simulink model "week1problem8"  (R2020a)
settings: Solver=VariableStepAuto  StartTime=0.0  StopTime=10.0  RelTol=1e-3
settings Model: Creator=Admin  LastModifiedBy=Admin

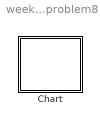
== system week1problem8 ==
  Chart : Stateflow chart  TreatAsAtomicUnit=on

== stateflow chart week1problem8/Chart ==
  state LiftOperation [parallel]
    entry:
    status=0;
    settings: executionOrder=1
    state LiftFunctionOn
      (history)
      state GroundFloor
        entry:
        status=1;
        during:
        CurrentFloor=0;
        FloorCheck(CurrentFloor);
        exit:
        status=0;
      state FirstFloor
        entry:
        status=1;
        during:
        CurrentFloor=1;
        FloorCheck(CurrentFloor);
        exit:
        status=0;
      state SecondFloor
        entry:
        status=1;
        during:
        CurrentFloor=2;
        FloorCheck(CurrentFloor);
        exit:
        status=0;
        after(1,sec);
      state ThirdFloor
        entry:
        status=1;
        during:
        CurrentFloor=3;
        FloorCheck(CurrentFloor);
        exit:
        status=0;
        after(1,sec);
      state FourthFloor
        entry:
        status=1
        during:
        CurrentFloor=4;
        FloorCheck(CurrentFloor);
        exit:
        status=0;
      state FifthFloor
        entry:
        status=1;
        during:
        CurrentFloor=5;
        FloorCheck(CurrentFloor);
        exit:
        status=0;
      (default) -> GroundFloor
      GroundFloor -> FirstFloor : up
      FirstFloor -> GroundFloor [order 2] : down
      FirstFloor -> SecondFloor [order 1] : up
      SecondFloor -> FirstFloor [order 2] : down
      SecondFloor -> ThirdFloor [order 1] : up
      ThirdFloor -> SecondFloor [order 2] : down
      ThirdFloor -> FourthFloor [order 1] : up
      FourthFloor -> ThirdFloor [order 1] : down
      FourthFloor -> FifthFloor [order 2] : up
      FifthFloor -> FourthFloor : down
    state LiftFunctionOff
      en:
      status=0;
    (default) -> LiftFunctionOn
    LiftFunctionOff -> LiftFunctionOn : [signal==0]
    LiftFunctionOn -> LiftFunctionOff : [signal==1]
  state Alarm [parallel]
    during:
    AlarmStatus = fire;
    FireStatusCheck(AlarmStatus);
    settings: executionOrder=2
